simulink model "gm_sampleModel61556_pp_34_1_sub"  (R2023b)
settings: Solver=VariableStepAuto  StartTime=0.0  StopTime=10.0  RelTol=1e-3
libraries: simulink x34
(part 2 of 2)

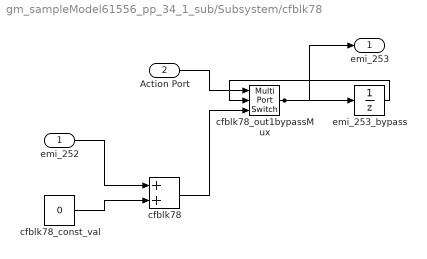
== system gm_sampleModel61556_pp_34_1_sub/Subsystem/cfblk78 ==
  emi_252 : Inport  OutDataTypeStr=uint8  PortDimensions=1  SampleTime=1
  Action Port : Inport  Port=2  OutDataTypeStr=boolean  SampleTime=1
  cfblk78 : Sum  OutDataTypeStr=uint8  AccumDataTypeStr=uint8  RndMeth=Nearest  SampleTime=1
  cfblk78_const_val : Constant  Value=0  VectorParams1D=off  OutDataTypeStr=uint8  SampleTime=1
  cfblk78_out1bypassMux : MultiPortSwitch  DataPortOrder=Zero-based contiguous  Inputs=2  zeroidx=on  OutDataTypeStr=uint8  SampleTime=1  SaturateOnIntegerOverflow=off  InputSameDT=off
  emi_253_bypass : UnitDelay  InitialCondition="fi(0,0,8,0,\"hex\",\"00\")"  SampleTime=1
  emi_253 : Outport  SampleTime=1  InitialOutput=0
  wires:
  Action Port/1 -> cfblk78_out1bypassMux/1
  emi_252/1 -> cfblk78/1
  cfblk78/1 -> cfblk78_out1bypassMux/3
  cfblk78_out1bypassMux/1 -> emi_253_bypass/1, emi_253/1
  emi_253_bypass/1 -> cfblk78_out1bypassMux/2
  cfblk78_const_val/1 -> cfblk78/2

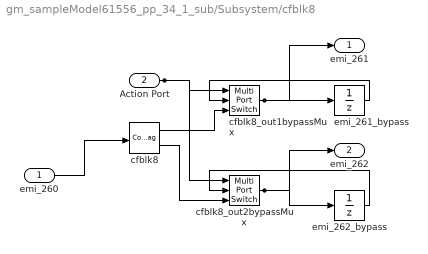
== system gm_sampleModel61556_pp_34_1_sub/Subsystem/cfblk8 ==
  emi_260 : Inport  OutDataTypeStr=uint8  PortDimensions=1  SampleTime=1
  Action Port : Inport  Port=2  OutDataTypeStr=boolean  SampleTime=1
  cfblk8 : ComplexToRealImag  SampleTime=1
  cfblk8_out1bypassMux : MultiPortSwitch  DataPortOrder=Zero-based contiguous  Inputs=2  zeroidx=on  OutDataTypeStr=uint8  SampleTime=1  SaturateOnIntegerOverflow=off  InputSameDT=off
  cfblk8_out2bypassMux : MultiPortSwitch  DataPortOrder=Zero-based contiguous  Inputs=2  zeroidx=on  OutDataTypeStr=uint8  SampleTime=1  SaturateOnIntegerOverflow=off  InputSameDT=off
  emi_261_bypass : UnitDelay  InitialCondition="fi(0,0,8,0,\"hex\",\"00\")"  SampleTime=1
  emi_262_bypass : UnitDelay  InitialCondition="fi(0,0,8,0,\"hex\",\"00\")"  SampleTime=1
  emi_261 : Outport  SampleTime=1  InitialOutput=0
  emi_262 : Outport  Port=2  SampleTime=1  InitialOutput=0
  wires:
  Action Port/1 -> cfblk8_out2bypassMux/1, cfblk8_out1bypassMux/1
  emi_260/1 -> cfblk8/1
  cfblk8/1 -> cfblk8_out1bypassMux/3
  cfblk8/2 -> cfblk8_out2bypassMux/3
  cfblk8_out1bypassMux/1 -> emi_261_bypass/1, emi_261/1
  emi_261_bypass/1 -> cfblk8_out1bypassMux/2
  cfblk8_out2bypassMux/1 -> emi_262_bypass/1, emi_262/1
  emi_262_bypass/1 -> cfblk8_out2bypassMux/2

== system gm_sampleModel61556_pp_34_1_sub/Subsystem/cfblk83 ==
  emi_269 : Inport  OutDataTypeStr=uint8  PortDimensions=1  SampleTime=1
  Action Port : Inport  Port=2  OutDataTypeStr=boolean  SampleTime=1
  Reshape : Reshape
  cfblk83_out1bypassMux : MultiPortSwitch  DataPortOrder=Zero-based contiguous  Inputs=2  zeroidx=on  OutDataTypeStr=uint8  SampleTime=1  SaturateOnIntegerOverflow=off  InputSameDT=off
  emi_270_bypass : UnitDelay  InitialCondition="fi(0,0,8,0,\"hex\",\"00\")"  SampleTime=1
  emi_270 : Outport  SampleTime=1  InitialOutput=0
  wires:
  Action Port/1 -> cfblk83_out1bypassMux/1
  emi_269/1 -> Reshape/1
  Reshape/1 -> cfblk83_out1bypassMux/3
  cfblk83_out1bypassMux/1 -> emi_270_bypass/1, emi_270/1
  emi_270_bypass/1 -> cfblk83_out1bypassMux/2

== system gm_sampleModel61556_pp_34_1_sub/Subsystem/cfblk84_inst ==
  in1 : Inport  OutDataTypeStr=uint8  SampleTime=1
  in2 : Inport  Port=2  OutDataTypeStr=uint8  SampleTime=1
  mul_cfblk84_dotp_mulcomp : Product  Inputs=**  OutDataTypeStr=uint8  SampleTime=1
  out1 : Outport  OutDataTypeStr=uint8  SampleTime=1
  wires:
  in1/1 -> mul_cfblk84_dotp_mulcomp/1
  in2/1 -> mul_cfblk84_dotp_mulcomp/2
  mul_cfblk84_dotp_mulcomp/1 -> out1/1

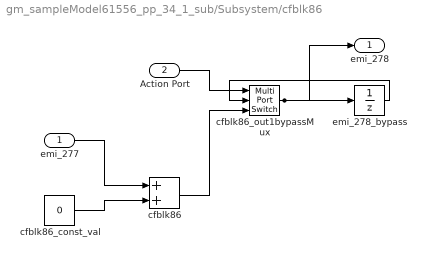
== system gm_sampleModel61556_pp_34_1_sub/Subsystem/cfblk86 ==
  emi_277 : Inport  OutDataTypeStr=uint8  PortDimensions=1  SampleTime=1
  Action Port : Inport  Port=2  OutDataTypeStr=boolean  SampleTime=1
  cfblk86 : Sum  OutDataTypeStr=uint8  AccumDataTypeStr=uint8  RndMeth=Nearest  SampleTime=1
  cfblk86_const_val : Constant  Value=0  VectorParams1D=off  OutDataTypeStr=uint8  SampleTime=1
  cfblk86_out1bypassMux : MultiPortSwitch  DataPortOrder=Zero-based contiguous  Inputs=2  zeroidx=on  OutDataTypeStr=uint8  SampleTime=1  SaturateOnIntegerOverflow=off  InputSameDT=off
  emi_278_bypass : UnitDelay  InitialCondition="fi(0,0,8,0,\"hex\",\"00\")"  SampleTime=1
  emi_278 : Outport  SampleTime=1  InitialOutput=0
  wires:
  Action Port/1 -> cfblk86_out1bypassMux/1
  emi_277/1 -> cfblk86/1
  cfblk86/1 -> cfblk86_out1bypassMux/3
  cfblk86_out1bypassMux/1 -> emi_278_bypass/1, emi_278/1
  emi_278_bypass/1 -> cfblk86_out1bypassMux/2
  cfblk86_const_val/1 -> cfblk86/2

== system gm_sampleModel61556_pp_34_1_sub/Subsystem/cfblk9 ==
  emi_293 : Inport  OutDataTypeStr=uint8  PortDimensions=1  SampleTime=1
  Action Port : Inport  Port=2  OutDataTypeStr=boolean  SampleTime=1
  cfblk9 : Abs  SampleTime=1  OutDataTypeStr=uint8  SaturateOnIntegerOverflow=off
  cfblk9_out1bypassMux : MultiPortSwitch  DataPortOrder=Zero-based contiguous  Inputs=2  zeroidx=on  OutDataTypeStr=uint8  SampleTime=1  SaturateOnIntegerOverflow=off  InputSameDT=off
  emi_294_bypass : UnitDelay  InitialCondition="fi(0,0,8,0,\"hex\",\"00\")"  SampleTime=1
  emi_294 : Outport  SampleTime=1  InitialOutput=0
  wires:
  Action Port/1 -> cfblk9_out1bypassMux/1
  emi_293/1 -> cfblk9/1
  cfblk9/1 -> cfblk9_out1bypassMux/3
  cfblk9_out1bypassMux/1 -> emi_294_bypass/1, emi_294/1
  emi_294_bypass/1 -> cfblk9_out1bypassMux/2

== system gm_sampleModel61556_pp_34_1_sub/Subsystem/cfblk90_inst ==
  in1 : Inport  OutDataTypeStr=uint8  SampleTime=1
  in2 : Inport  Port=2  OutDataTypeStr=uint8  SampleTime=1
  mul_cfblk90_dotp_mulcomp : Product  Inputs=**  OutDataTypeStr=uint8  SampleTime=1
  out1 : Outport  OutDataTypeStr=uint8  SampleTime=1
  wires:
  in1/1 -> mul_cfblk90_dotp_mulcomp/1
  in2/1 -> mul_cfblk90_dotp_mulcomp/2
  mul_cfblk90_dotp_mulcomp/1 -> out1/1

== system gm_sampleModel61556_pp_34_1_sub/Subsystem/cfblk91 ==
  emi_301 : Inport  OutDataTypeStr=uint8  PortDimensions=1  SampleTime=1
  Action Port : Inport  Port=2  OutDataTypeStr=boolean  SampleTime=1
  cfblk91 : Abs  SampleTime=1  OutDataTypeStr=uint8  SaturateOnIntegerOverflow=off
  cfblk91_out1bypassMux : MultiPortSwitch  DataPortOrder=Zero-based contiguous  Inputs=2  zeroidx=on  OutDataTypeStr=uint8  SampleTime=1  SaturateOnIntegerOverflow=off  InputSameDT=off
  emi_302_bypass : UnitDelay  InitialCondition="fi(0,0,8,0,\"hex\",\"00\")"  SampleTime=1
  emi_302 : Outport  SampleTime=1  InitialOutput=0
  wires:
  Action Port/1 -> cfblk91_out1bypassMux/1
  emi_301/1 -> cfblk91/1
  cfblk91/1 -> cfblk91_out1bypassMux/3
  cfblk91_out1bypassMux/1 -> emi_302_bypass/1, emi_302/1
  emi_302_bypass/1 -> cfblk91_out1bypassMux/2

== system gm_sampleModel61556_pp_34_1_sub/Subsystem/cfblk93_inst ==
  in1 : Inport  OutDataTypeStr=uint8  SampleTime=1
  in2 : Inport  Port=2  OutDataTypeStr=uint8  SampleTime=1
  mul_cfblk93_dotp_mulcomp : Product  Inputs=**  OutDataTypeStr=uint8  SampleTime=1
  out1 : Outport  OutDataTypeStr=uint8  SampleTime=1
  wires:
  in1/1 -> mul_cfblk93_dotp_mulcomp/1
  in2/1 -> mul_cfblk93_dotp_mulcomp/2
  mul_cfblk93_dotp_mulcomp/1 -> out1/1

== system gm_sampleModel61556_pp_34_1_sub/Subsystem/cfblk96 ==
  emi_309 : Inport  OutDataTypeStr=uint8  PortDimensions=1  SampleTime=1
  Action Port : Inport  Port=2  OutDataTypeStr=boolean  SampleTime=1
  cfblk96 : MinMax
  cfblk96_out1bypassMux : MultiPortSwitch  DataPortOrder=Zero-based contiguous  Inputs=2  zeroidx=on  OutDataTypeStr=uint8  SampleTime=1  SaturateOnIntegerOverflow=off  InputSameDT=off
  emi_310_bypass : UnitDelay  InitialCondition="fi(0,0,8,0,\"hex\",\"00\")"  SampleTime=1
  emi_310 : Outport  SampleTime=1  InitialOutput=0
  wires:
  Action Port/1 -> cfblk96_out1bypassMux/1
  emi_309/1 -> cfblk96/1
  cfblk96/1 -> cfblk96_out1bypassMux/3
  cfblk96_out1bypassMux/1 -> emi_310_bypass/1, emi_310/1
  emi_310_bypass/1 -> cfblk96_out1bypassMux/2

== system gm_sampleModel61556_pp_34_1_sub/Subsystem/cfblk111/cfblk111 ==
  u : Inport  OutDataTypeStr=uint8  SampleTime=1
  FixPt Constant : Constant  DisableCoverage=on  OutDataTypeStr=Inherit: Inherit via back propagation  SampleTime=-1
  FixPt Data Type Duplicate : DataTypeDuplicate  DisableCoverage=on  NumInputPorts=3
  FixPt Sum1 : Sum  OutDataTypeStr=Inherit: Inherit via back propagation  InputSameDT=on  LockScale=on
  y : Outport  SampleTime=1  InitialOutput=0
  wires:
  u/1 -> FixPt Sum1/1, FixPt Data Type Duplicate/2
  FixPt Constant/1 -> FixPt Sum1/2, FixPt Data Type Duplicate/3
  FixPt Sum1/1 -> FixPt Data Type Duplicate/1, y/1

== system gm_sampleModel61556_pp_34_1_sub/Subsystem/cfblk153/cfblk153 ==
  u : Inport  OutDataTypeStr=uint8  SampleTime=1
  FixPt Constant : Constant  DisableCoverage=on  OutDataTypeStr=Inherit: Inherit via back propagation  SampleTime=-1
  FixPt Data Type Duplicate : DataTypeDuplicate  DisableCoverage=on  NumInputPorts=3
  FixPt Sum1 : Sum  OutDataTypeStr=Inherit: Inherit via back propagation  InputSameDT=on  LockScale=on
  y : Outport  SampleTime=1  InitialOutput=0
  wires:
  u/1 -> FixPt Sum1/1, FixPt Data Type Duplicate/2
  FixPt Constant/1 -> FixPt Sum1/2, FixPt Data Type Duplicate/3
  FixPt Sum1/1 -> FixPt Data Type Duplicate/1, y/1

== system gm_sampleModel61556_pp_34_1_sub/Subsystem/cfblk191/cfblk191 ==
  in0 : Inport  OutDataTypeStr=uint8  SampleTime=1
  Action Port_out2 : EnablePort  OutDataTypeStr=boolean
  cfblk191 : Delay  DelayLength=double(2)  InitialCondition=0
  out0 : Outport  OutDataTypeStr=uint8  SampleTime=1  InitialOutput=0
  wires:
  cfblk191/1 -> out0/1
  in0/1 -> cfblk191/1

== system gm_sampleModel61556_pp_34_1_sub/Subsystem/cfblk2/Nonnegative ==
  u : Inport  OutDataTypeStr=uint8  SampleTime=1
  Compare : RelationalOperator  OutDataTypeStr=boolean  ZeroCross=off
  Constant : Constant  DisableCoverage=on  Value=0  OutDataTypeStr=Inherit: Inherit via back propagation  SampleTime=-1  PreserveConstantTs=on
  y : Outport  SampleTime=1
  wires:
  u/1 -> Compare/1
  Compare/1 -> y/1
  Constant/1 -> Compare/2

== system gm_sampleModel61556_pp_34_1_sub/Subsystem/cfblk4/cfblk4 ==
  note: U(k)
  note: Edge
  U : Inport  OutDataTypeStr=uint8  SampleTime=1
  Action Port_out2 : Inport  Port=2  OutDataTypeStr=boolean  SampleTime=1
  Delay Input1 : Subsystem
      settings: MinAlgLoopOccurrences=on
  FixPt Relational Operator : RelationalOperator  Operator=>  OutDataTypeStr=fixdt(0,8,0)  SampleTime=1  InputSameDT=off
  Positive : Subsystem  mask(Compare To Zero){relop=>, OutDataTypeStr=boolean, ZeroCross=off}
      mask prompts: relop "Simulink:masks:Operator_MP"; OutDataTypeStr "Simulink:masks:OutputDataType_MP"; ZeroCross "Simulink:masks:EnableZerocrossingDetection_MP"
      mask help: Simulink:masks:CompareToZero_MD
      mask TypeOptions relop: == | ~= | < | <= | >= | >
      mask TypeOptions OutDataTypeStr: Simulink:masks:uint8 | Simulink:masks:boolean
      mask Callback ZeroCross: sl('zeroCrossEnable', gcbh);
      mask Display: disp([relop,' 0'])
  Y : Outport  SampleTime=1  InitialOutput=0
  wires:
  U/1 -> Positive/1(u)
  Delay Input1/1(out0) -> FixPt Relational Operator/2
  FixPt Relational Operator/1 -> Y/1
  Positive/1(y) -> FixPt Relational Operator/1, Delay Input1/1(in0)
  Action Port_out2/1 -> Delay Input1/Enable

== system gm_sampleModel61556_pp_34_1_sub/Subsystem/cfblk4/cfblk4/Delay Input1 ==
  in0 : Inport  OutDataTypeStr=boolean  SampleTime=1
  Action Port_out2 : EnablePort  OutDataTypeStr=boolean
  Delay Input1 : UnitDelay  SampleTime=1
  out0 : Outport  OutDataTypeStr=boolean  SampleTime=1  InitialOutput=0
  wires:
  Delay Input1/1 -> out0/1
  in0/1 -> Delay Input1/1

== system gm_sampleModel61556_pp_34_1_sub/Subsystem/cfblk4/cfblk4/Positive ==
  u : Inport  OutDataTypeStr=uint8  SampleTime=1
  Compare : RelationalOperator  Operator=>  OutDataTypeStr=boolean  SampleTime=1
  Constant : Constant  Value=0  OutDataTypeStr=uint8  SampleTime=1
  y : Outport  SampleTime=1  InitialOutput=0
  wires:
  u/1 -> Compare/1
  Compare/1 -> y/1
  Constant/1 -> Compare/2
